simulink library "TankPressure_Lib"  (R2021a)
settings: Solver=VariableStepAuto  StartTime=0.0  StopTime=10.0  RelTol=1e-3
settings Model: Creator=Christian  LastModifiedBy=Christian
settings SolverCC: AlgebraicLoopSolver=TrustRegion
settings DebuggingCC: SFMachineParentedDataDiag=warning

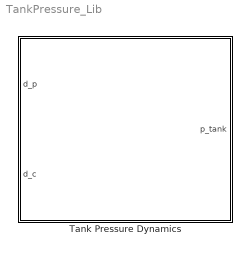
== system TankPressure_Lib ==
  Tank Pressure Dynamics : Subsystem  mask{p_0=0, A=0, B_producer=0, B_consumer=0, Ts=0}
      mask prompts: p_0 "Initial pressure"; A "State Matrix"; B_producer "Input matrix"; B_consumer "Disturbance matrix"; Ts "Sample time"

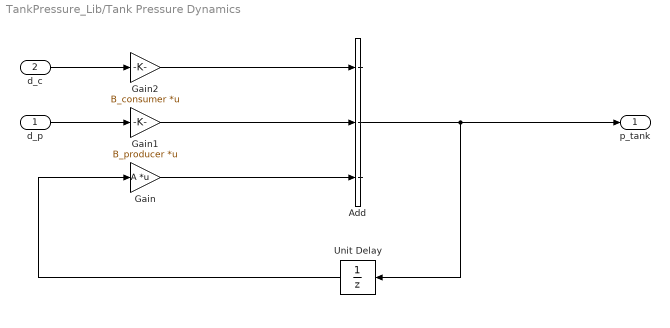
== system TankPressure_Lib/Tank Pressure Dynamics ==
  d_p : Inport  PortDimensions=[2 1]
  d_c : Inport  Port=2  PortDimensions=[2 1]
  Add : Sum  Inputs=+++
  Gain : Gain  Gain=A  Multiplication=Matrix(K*u)
  Gain1 : Gain  Gain=B_producer  Multiplication=Matrix(K*u)
  Gain2 : Gain  Gain=B_consumer  Multiplication=Matrix(K*u)
  Unit Delay : UnitDelay  InitialCondition=p_0  SampleTime=Ts  HasFrameUpgradeWarning=on
  p_tank : Outport
  wires:
  Add/1 -> p_tank/1, Unit Delay/1
  Gain1/1 -> Add/2
  d_p/1 -> Gain1/1
  Unit Delay/1 -> Gain/1
  Gain/1 -> Add/3
  Gain2/1 -> Add/1
  d_c/1 -> Gain2/1
